simulink model "sir"  (R2020b)
settings: Solver=VariableStepAuto  StartTime=0.0  StopTime=10.0  RelTol=1e-3
values from neighbouring files (symbols this model uses):
  a = 0.44    [sir.m]
  I0 = 1    [sir.m]
  r = 2.18*1e-3    (= 0.00218)    [sir.m]
  R0 = 0    [sir.m]
  S0 = 762    [sir.m]
settings Model: Creator=Admin  LastModifiedBy=Admin

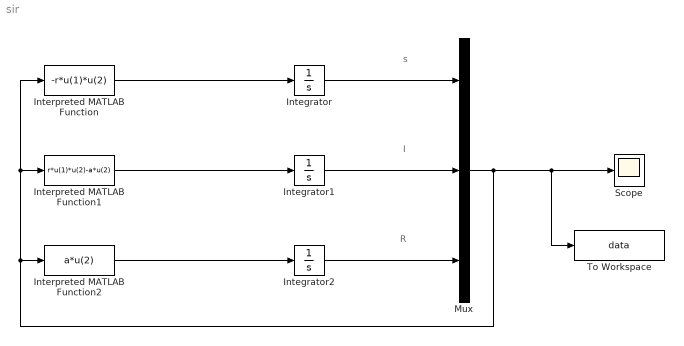
== system sir ==
  note: R
  note: I
  note: s
  Integrator : Integrator  InitialCondition=S0
  Integrator1 : Integrator  InitialCondition=I0
  Integrator2 : Integrator  InitialCondition=R0
  Interpreted MATLAB Function : MATLABFcn  MATLABFcn=-r*u(1)*u(2)  OutputDimensions=1
  Interpreted MATLAB Function1 : MATLABFcn  MATLABFcn=r*u(1)*u(2)-a*u(2)  OutputDimensions=1
  Interpreted MATLAB Function2 : MATLABFcn  MATLABFcn=a*u(2)
  Mux : Mux  Inputs=3
  Scope : Scope
  To Workspace : ToWorkspace  VariableName=data  SaveFormat=Structure With Time  SampleTime=-1
  wires:
  Integrator/1 -> Mux/1
  Integrator1/1 -> Mux/2
  Integrator2/1 -> Mux/3
  Interpreted MATLAB Function2/1 -> Integrator2/1
  Interpreted MATLAB Function1/1 -> Integrator1/1
  Interpreted MATLAB Function/1 -> Integrator/1
  Mux/1 -> To Workspace/1, Scope/1, Interpreted MATLAB Function/1, Interpreted MATLAB Function1/1, Interpreted MATLAB Function2/1
